simulink model "sistema"  (R2015a)
settings: Solver=ode45  StartTime=0.0  StopTime=10.0  RelTol=1e-3
values from neighbouring files (symbols this model uses):
  Bs = 11    [init_model.m]
undefined symbols (not defined in the file or in its folder): A, As, B, C, Cs, D, De, Ds, Ke, Me
libraries: simulink x1
settings Model: Creator=enrico-giordano  LastModifiedBy=enrico-giordano

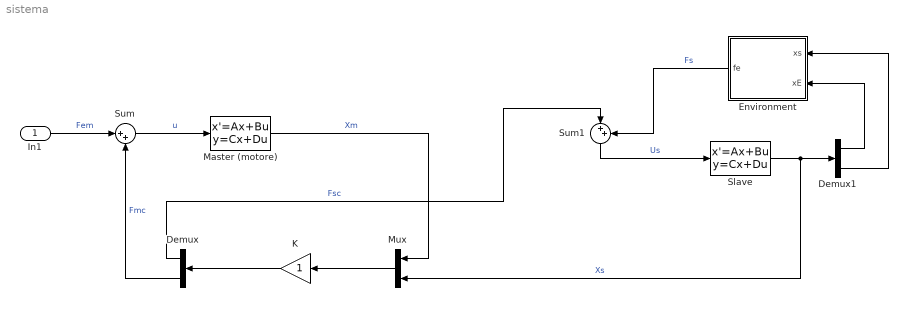
== system sistema ==
  In1 : Inport
  Demux : Demux  Outputs=2
  Demux1 : Demux  Outputs=2
  Environment : Subsystem
  K : Gain
  Master (motore) : StateSpace  A=A  B=B  C=C  D=D  X0=0
  Mux : Mux  Inputs=2
  Slave : StateSpace  A=As  B=Bs  C=Cs  D=Ds  X0=0
  Sum : Sum  Inputs=|++
  Sum1 : Sum  Inputs=|++
  wires:
  Sum/1 -> Master (motore)/1  "u"
  In1/1 -> Sum/1  "Fem"
  Demux/2 -> Sum/2  "Fmc"
  K/1 -> Demux/1
  Mux/1 -> K/1
  Master (motore)/1 -> Mux/1  "Xm"
  Demux/1 -> Sum1/1  "Fsc"
  Sum1/1 -> Slave/1  "Us"
  Environment/1(fe) -> Sum1/2  "Fs"
  Demux1/1 -> Environment/2(xE)
  Demux1/2 -> Environment/1(xs)
  Slave/1 -> Demux1/1, Mux/2  "Xs"

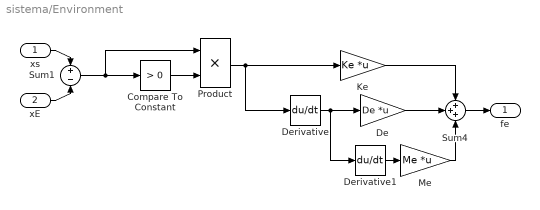
== system sistema/Environment ==
  xs : Inport
  xE : Inport  Port=2
  Compare To Constant : simulink/Logic and Bit Operations/Compare To Constant  SystemSampleTime=-1  relop=>  const=0  LogicOutDataTypeMode=uint8  ZeroCross=off
  De : Gain  Gain=De  Multiplication=Matrix(K*u)
  Derivative : Derivative
  Derivative1 : Derivative
  Ke : Gain  Gain=Ke  Multiplication=Matrix(K*u)
  Me : Gain  Gain=Me  Multiplication=Matrix(K*u)
  Product : Product  RndMeth=Zero
  Sum1 : Sum  Inputs=+|-
  Sum4 : Sum  Inputs=+++
  fe : Outport
  wires:
  Compare To Constant/1 -> Product/2
  Sum1/1 -> Compare To Constant/1, Product/1
  Product/1 -> Ke/1, Derivative/1
  Derivative/1 -> De/1, Derivative1/1
  Derivative1/1 -> Me/1
  Ke/1 -> Sum4/1
  De/1 -> Sum4/2
  Me/1 -> Sum4/3
  xs/1 -> Sum1/1
  xE/1 -> Sum1/2
  Sum4/1 -> fe/1
